simulink model "Quaternions_Method_main"  (R2021b)
settings: Solver=ode4  StartTime=0.0  StopTime=Time  FixedStep=1e-2  RelTol=1e-13  AbsTol=1e-8
values from neighbouring files (symbols this model uses):
  a = 8.6251e+06    (= 8625100)    [Main.m]
  c = 299792*10^3    (= 299792000)    [Main.m]
  e = 0.1195    [Main.m]
  f_mag = 18    [Main.m]
  H_0 = sqrt((g_1_0)^2 + (g_1_1)^2 + (h_1_1)^2)    [Main.m]
  i = 0.3815    [Main.m]
  MB = [2000; 0.3; 1; 0.12].*1e-2    [Main.m]
  muP = G*Mt    (= 398527110340000)    [Main.m]
  omega_0 = [om_x, om_y, om_z]    [Main.m]
  p_acc = 0.5    [Main.m]
  RD = 0.1*ones(1,10)    [Main.m]
  RS_MB = 0.5    [Main.m]
  RS_SP = 0.1    [Main.m]
  SP = [2000; 0.3; 1; 0.12].*1e-2    [Main.m]
  theta0 = 0    [Main.m]
  w_E = (2*pi)/(24*3600)    (= 7.27220521664e-05)    [Main.m]
undefined symbols (not defined in the file or in its folder): A_BN_0, A_rw, A_rw_star, k1, k2, magnitude, mr, sig_b, sig_n, T, t_sample
libraries: matrix_library x15, vrlib x8, simulink x2, simulink_extras x1
(part 3 of 5)

== system Quaternions_Method_main/Enviroment/Magnetic torque /Magnetic torque in body frame/Direction of M field ==
  Clock : Clock
  Constant : Constant  Value=eps
  Constant1 : Constant  Value=w_E
  Mux : Mux  Inputs=3
  Product : Product
  Product1 : Product
  Product2 : Product
  Reshape : Reshape  OutputDimensionality=Column vector (2-D)
  Trigonometric Function : Trigonometry
  Trigonometric Function1 : Trigonometry  Operator=cos
  Trigonometric Function2 : Trigonometry  Operator=cos
  Trigonometric Function3 : Trigonometry
  m_vect : Outport
  wires:
  Constant1/1 -> Product/1
  Clock/1 -> Product/2
  Constant/1 -> Trigonometric Function2/1, Trigonometric Function/1
  Product/1 -> Trigonometric Function3/1, Trigonometric Function1/1
  Trigonometric Function/1 -> Product2/1, Product1/1
  Trigonometric Function1/1 -> Product1/2
  Trigonometric Function3/1 -> Product2/2
  Product1/1 -> Mux/1
  Product2/1 -> Mux/2
  Trigonometric Function2/1 -> Mux/3
  Mux/1 -> Reshape/1
  Reshape/1 -> m_vect/1

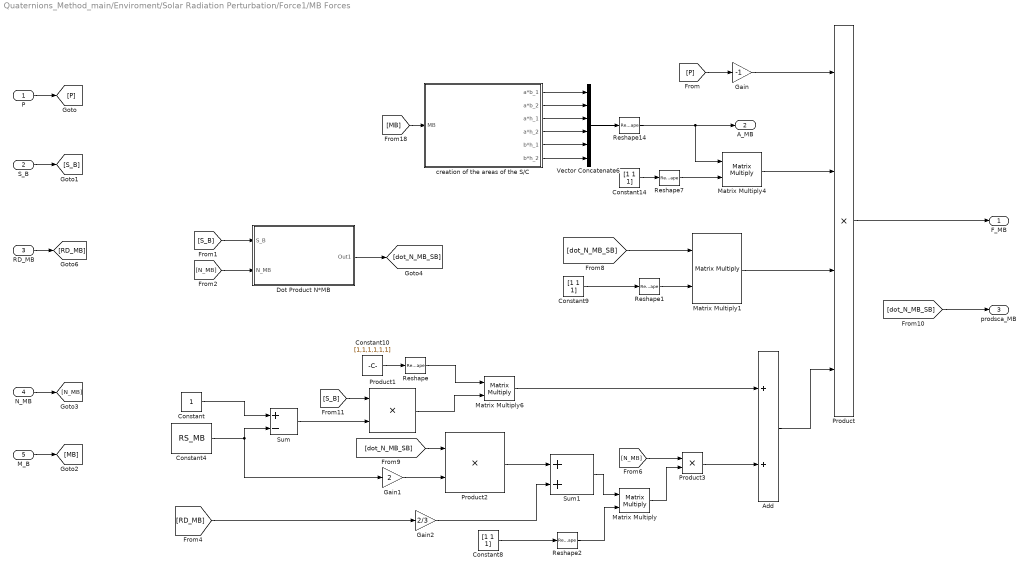
== system Quaternions_Method_main/Enviroment/Solar Radiation Perturbation/Force1/MB Forces ==
  P : Inport
  S_B : Inport  Port=2
  RD_MB : Inport  Port=3
  N_MB : Inport  Port=4
  M_B : Inport  Port=5
  Add : Sum
  Constant : Constant
  Constant10 : Constant  Value=[1,1,1,1,1,1]
  Constant14 : Constant  Value=[1 1 1]
  Constant4 : Constant  Value=RS_MB
  Constant8 : Constant  Value=[1 1 1]
  Constant9 : Constant  Value=[1 1 1]
  Dot Product N*MB : Subsystem
  Gain : Gain  Gain=-1
  Gain1 : Gain  Gain=2
  Gain2 : Gain  Gain=2/3
  Matrix Multiply{,1,4,6} (4 alike) : Product  Multiplication=Matrix(*)
  Product : Product  Inputs=4
  Product1 : Product
  Product2 : Product
  Product3 : Product
  Reshape : Reshape  OutputDimensionality=Column vector (2-D)
  Reshape1 : Reshape  OutputDimensionality=Row vector (2-D)
  Reshape14 : Reshape  OutputDimensionality=Column vector (2-D)
  Reshape2 : Reshape  OutputDimensionality=Row vector (2-D)
  Reshape7 : Reshape  OutputDimensionality=Row vector (2-D)
  Sum : Sum  Inputs=+-
  Sum1 : Sum
  Vector Concatenate6 : Concatenate  NumInputs=6
  creation of the areas of the S/C : Subsystem
  F_MB : Outport
  A_MB : Outport  Port=2
  prodsca_MB : Outport  Port=3
  wires:
  Constant4/1 -> Sum/2, Gain1/1
  Matrix Multiply6/1 -> Add/1
  Vector Concatenate6/1 -> Reshape14/1
  Constant9/1 -> Reshape1/1
  Reshape1/1 -> Matrix Multiply1/2
  Constant/1 -> Sum/1
  Reshape2/1 -> Matrix Multiply/2
  Gain/1 -> Product/1
  [S_B] -> Product1/1
  Sum/1 -> Product1/2
  creation of the areas of the S/C/1(a*b_1) -> Vector Concatenate6/1
  Add/1 -> Product/4
  Constant8/1 -> Reshape2/1
  Gain2/1 -> Sum1/2
  [dot_N_MB_SB] -> prodsca_MB/1
  [RD_MB] -> Gain2/1
  creation of the areas of the S/C/2(a*b_2) -> Vector Concatenate6/2
  [P] -> Gain/1
  Product2/1 -> Sum1/1
  Matrix Multiply/1 -> Product3/2
  [dot_N_MB_SB] -> Matrix Multiply1/1
  Matrix Multiply4/1 -> Product/2
  Reshape14/1 -> A_MB/1, Matrix Multiply4/1
  Matrix Multiply1/1 -> Product/3
  Gain1/1 -> Product2/2
  Sum1/1 -> Matrix Multiply/1
  creation of the areas of the S/C/4(a*h_2) -> Vector Concatenate6/4
  [dot_N_MB_SB] -> Product2/1
  creation of the areas of the S/C/5(b*h_1) -> Vector Concatenate6/5
  creation of the areas of the S/C/6(b*h_2) -> Vector Concatenate6/6
  Product1/1 -> Matrix Multiply6/2
  creation of the areas of the S/C/3(a*h_1) -> Vector Concatenate6/3
  [MB] -> creation of the areas of the S/C/1(MB)
  Constant14/1 -> Reshape7/1
  Product/1 -> F_MB/1
  Reshape7/1 -> Matrix Multiply4/2
  Product3/1 -> Add/2
  Constant10/1 -> Reshape/1
  Reshape/1 -> Matrix Multiply6/1
  [N_MB] -> Product3/1
  Dot Product N*MB/1(Out1) -> [dot_N_MB_SB]
  S_B/1 -> [S_B]
  RD_MB/1 -> [RD_MB]
  P/1 -> [P]
  N_MB/1 -> [N_MB]
  M_B/1 -> [MB]
  [S_B] -> Dot Product N*MB/1(S_B)
  [N_MB] -> Dot Product N*MB/2(N_MB)

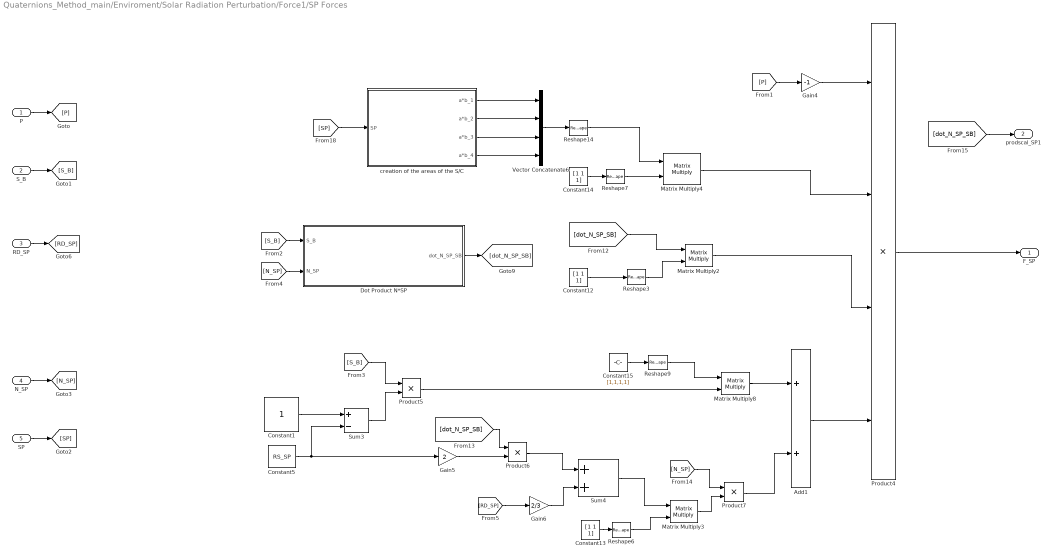
== system Quaternions_Method_main/Enviroment/Solar Radiation Perturbation/Force1/SP Forces ==
  P : Inport
  S_B : Inport  Port=2
  RD_SP : Inport  Port=3
  N_SP : Inport  Port=4
  SP : Inport  Port=5
  Add1 : Sum
  Constant1 : Constant
  Constant12 : Constant  Value=[1 1 1]
  Constant13 : Constant  Value=[1 1 1]
  Constant14 : Constant  Value=[1 1 1]
  Constant15 : Constant  Value=[1,1,1,1]
  Constant5 : Constant  Value=RS_SP
  Dot Product N*SP : Subsystem
  Gain4 : Gain  Gain=-1
  Gain5 : Gain  Gain=2
  Gain6 : Gain  Gain=2/3
  Matrix Multiply{2..4,8} (4 alike) : Product  Multiplication=Matrix(*)
  Product4 : Product  Inputs=4
  Product5 : Product
  Product6 : Product
  Product7 : Product
  Reshape14 : Reshape  OutputDimensionality=Column vector (2-D)
  Reshape3 : Reshape  OutputDimensionality=Row vector (2-D)
  Reshape6 : Reshape  OutputDimensionality=Row vector (2-D)
  Reshape7 : Reshape  OutputDimensionality=Row vector (2-D)
  Reshape9 : Reshape  OutputDimensionality=Column vector (2-D)
  Sum3 : Sum  Inputs=+-
  Sum4 : Sum
  Vector Concatenate6 : Concatenate  NumInputs=4
  creation of the areas of the S/C : Subsystem
  F_SP : Outport
  prodscal_SP1 : Outport  Port=2
  wires:
  Sum3/1 -> Product5/2
  Reshape3/1 -> Matrix Multiply2/2
  Constant13/1 -> Reshape6/1
  Gain4/1 -> Product4/1
  Product6/1 -> Sum4/1
  Constant12/1 -> Reshape3/1
  [S_B] -> Product5/1
  [P] -> Gain4/1
  Gain6/1 -> Sum4/2
  [RD_SP] -> Gain6/1
  [N_SP] -> Product7/1
  Constant1/1 -> Sum3/1
  Constant15/1 -> Reshape9/1
  Sum4/1 -> Matrix Multiply3/1
  Product4/1 -> F_SP/1
  Constant5/1 -> Gain5/1, Sum3/2
  [dot_N_SP_SB] -> Matrix Multiply2/1
  Reshape6/1 -> Matrix Multiply3/2
  Product5/1 -> Matrix Multiply8/2
  Matrix Multiply3/1 -> Product7/2
  Gain5/1 -> Product6/2
  Matrix Multiply2/1 -> Product4/3
  Reshape9/1 -> Matrix Multiply8/1
  Product7/1 -> Add1/2
  [dot_N_SP_SB] -> Product6/1
  Add1/1 -> Product4/4
  [dot_N_SP_SB] -> prodscal_SP1/1
  Matrix Multiply8/1 -> Add1/1
  S_B/1 -> [S_B]
  N_SP/1 -> [N_SP]
  P/1 -> [P]
  SP/1 -> [SP]
  RD_SP/1 -> [RD_SP]
  Matrix Multiply4/1 -> Product4/2
  Vector Concatenate6/1 -> Reshape14/1
  Reshape14/1 -> Matrix Multiply4/1
  Constant14/1 -> Reshape7/1
  [SP] -> creation of the areas of the S/C/1(SP)
  Reshape7/1 -> Matrix Multiply4/2
  creation of the areas of the S/C/1(a*b_1) -> Vector Concatenate6/1
  creation of the areas of the S/C/2(a*b_2) -> Vector Concatenate6/2
  creation of the areas of the S/C/3(a*b_3) -> Vector Concatenate6/3
  creation of the areas of the S/C/4(a*b_4) -> Vector Concatenate6/4
  [S_B] -> Dot Product N*SP/1(S_B)
  [N_SP] -> Dot Product N*SP/2(N_SP)
  Dot Product N*SP/1(dot_N_SP_SB) -> [dot_N_SP_SB]

== system Quaternions_Method_main/Enviroment/Solar Radiation Perturbation/Sum forces/determine highlighted area ==
  note: matrice che ha per colonne i vettori distanza tra il CM del MB e i centri geom delle aree illuminate dal sole
  MB : Inport
  A_MB : Inport  Port=2
  prodscal_MB(tra norm e sun direction) : Inport  Port=3
  Demux1 : Demux  Outputs=6
  Demux2 : Demux  Outputs=6
  If : If  NumInputs=2  IfExpression=u1>0  ElseIfExpressions=u2>0
  If Action Subsystem : Subsystem  TreatAsAtomicUnit=on
  If Action Subsystem1 : Subsystem  TreatAsAtomicUnit=on
  If Action Subsystem2 : Subsystem  TreatAsAtomicUnit=on
  If Action Subsystem3 : Subsystem  TreatAsAtomicUnit=on
  If Action Subsystem4 : Subsystem  TreatAsAtomicUnit=on
  If Action Subsystem5 : Subsystem  TreatAsAtomicUnit=on
  If Action Subsystem6 : Subsystem  TreatAsAtomicUnit=on
  If Action Subsystem7 : Subsystem  TreatAsAtomicUnit=on
  If Action Subsystem8 : Subsystem  TreatAsAtomicUnit=on
  If1 : If  NumInputs=2  IfExpression=u1>0  ElseIfExpressions=u2>0
  If2 : If  NumInputs=2  IfExpression=u1>0  ElseIfExpressions=u2>0
  Merge : Merge  Inputs=3
  Merge1 : Merge  Inputs=3
  Merge2 : Merge  Inputs=3
  Mux : Mux  Inputs=3
  Product{10..15} (6 alike) : Product
  Reshape : Reshape  OutputDimensionality=Column vector (2-D)
  Reshape1 : Reshape  OutputDimensionality=Column vector (2-D)
  "creazione della matrice che ha per colonne i vettori distanza tra il CM del MB e i centri geom delle aree illuminate dal sole " : Subsystem
  distance matrix : Outport
  wires:
  Reshape/1 -> Demux2/1
  prodscal_MB(tra norm e sun direction)/1 -> Reshape/1
  Demux2/1 -> Product15/2  "x"
  Demux2/2 -> Product13/2  "y"
  Demux2/3 -> Product12/2  "z"
  Demux2/4 -> Product11/2  "-x"
  Demux2/5 -> Product10/2  "-y"
  Demux2/6 -> Product14/2  "-z"
  Demux1/1 -> Product12/1
  Mux/1 -> Reshape1/1
  Product15/1 -> If Action Subsystem/1(In1), If/1  "x"
  If/1 -> If Action Subsystem/Action
  Reshape1/1 -> "creazione della matrice che ha per colonne i vettori distanza tra il CM del MB e i centri geom delle aree illuminate dal sole "/2(A_vect)  "Areas_vect = vettore contenente le aree nelle direzioni x, y, z, -x, -y, -z"
  "creazione della matrice che ha per colonne i vettori distanza tra il CM del MB e i centri geom delle aree illuminate dal sole "/1(distance matrix) -> distance matrix/1
  A_MB/1 -> Demux1/1
  Demux1/2 -> Product14/1
  Demux1/3 -> Product13/1
  Demux1/4 -> Product10/1
  Demux1/5 -> Product15/1
  Demux1/6 -> Product11/1
  If/2 -> If Action Subsystem1/Action
  Product11/1 -> If Action Subsystem1/1(In1), If/2  "-x"
  If1/2 -> If Action Subsystem4/Action
  If1/3 -> If Action Subsystem5/Action
  If1/1 -> If Action Subsystem3/Action
  Product10/1 -> If Action Subsystem4/1(In1), If1/2  "-y"
  Product13/1 -> If Action Subsystem3/1(In1), If1/1  "y"
  If2/2 -> If Action Subsystem7/Action
  If2/3 -> If Action Subsystem8/Action
  If2/1 -> If Action Subsystem6/Action
  Product12/1 -> If Action Subsystem6/1(In1), If2/1  "z"
  Product14/1 -> If Action Subsystem7/1(In1), If2/2  "-z"
  Merge/1 -> Mux/2
  Merge2/1 -> Mux/3
  Merge1/1 -> Mux/1
  If Action Subsystem8/1(Out1) -> Merge2/3
  If Action Subsystem7/1(Out1) -> Merge2/2
  If Action Subsystem6/1(Out1) -> Merge2/1
  If Action Subsystem5/1(Out1) -> Merge/3
  If Action Subsystem4/1(Out1) -> Merge/2
  MB/1 -> "creazione della matrice che ha per colonne i vettori distanza tra il CM del MB e i centri geom delle aree illuminate dal sole "/1(MB)
  If Action Subsystem/1(Out1) -> Merge1/1
  If Action Subsystem1/1(Out1) -> Merge1/2
  If/3 -> If Action Subsystem2/Action
  If Action Subsystem2/1(Out1) -> Merge1/3
  If Action Subsystem3/1(Out1) -> Merge/1

== system Quaternions_Method_main/Enviroment/Solar Radiation Perturbation/Sum forces/determine highlighted area1 ==
  prodscal_SP(tra norm e sun direction) : Inport
  Demux2 : Demux
  If : If  NumInputs=2  IfExpression=u1>0  ElseIfExpressions=u2>0
  If Action Subsystem : Subsystem  TreatAsAtomicUnit=on
  If Action Subsystem1 : Subsystem  TreatAsAtomicUnit=on
  If Action Subsystem2 : Subsystem  TreatAsAtomicUnit=on
  If Action Subsystem3 : Subsystem  TreatAsAtomicUnit=on
  If Action Subsystem4 : Subsystem  TreatAsAtomicUnit=on
  If Action Subsystem5 : Subsystem  TreatAsAtomicUnit=on
  If1 : If  NumInputs=2  IfExpression=u1>0  ElseIfExpressions=u2>0
  Merge : Merge  Inputs=3
  Merge1 : Merge  Inputs=3
  Mux : Mux  Inputs=2
  Reshape : Reshape  OutputDimensionality=Column vector (2-D)
  Reshape1 : Reshape  OutputDimensionality=Column vector (2-D)
  face illuminated : Outport
  wires:
  If Action Subsystem2/1(Out1) -> Merge/3
  If/3 -> If Action Subsystem2/Action
  Merge/1 -> Mux/1
  Demux2/1 -> If/1  "y_1"
  Mux/1 -> Reshape1/1
  Demux2/2 -> If/2  "-y_1"
  prodscal_SP(tra norm e sun direction)/1 -> Reshape/1
  Reshape/1 -> Demux2/1
  Demux2/3 -> If1/1  "y_2"
  Demux2/4 -> If1/2  "-y_2"
  Merge1/1 -> Mux/2
  Reshape1/1 -> face illuminated/1
  If/1 -> If Action Subsystem/Action
  If Action Subsystem/1(Out1) -> Merge/1
  If/2 -> If Action Subsystem1/Action
  If Action Subsystem1/1(Out1) -> Merge/2
  If Action Subsystem4/1(Out1) -> Merge1/2
  If1/2 -> If Action Subsystem4/Action
  If1/1 -> If Action Subsystem3/Action
  If1/3 -> If Action Subsystem5/Action
  If Action Subsystem5/1(Out1) -> Merge1/3
  If Action Subsystem3/1(Out1) -> Merge1/1

== system Quaternions_Method_main/Kinematics1/Creazione quaternione/DCM to quaternion/Case 1 ==
  A11 : Inport
  A22 : Inport  Port=2
  A33 : Inport  Port=3
  Add : Sum  Inputs=++--
  Constant : Constant
  Gain : Gain  Gain=1/2
  Sqrt : Sqrt  SaturateOnIntegerOverflow=on
  q1 : Outport
  wires:
  A22/1 -> Add/3
  A11/1 -> Add/2
  A33/1 -> Add/4
  Constant/1 -> Add/1
  Add/1 -> Sqrt/1
  Sqrt/1 -> Gain/1
  Gain/1 -> q1/1

== system Quaternions_Method_main/Kinematics1/Creazione quaternione/DCM to quaternion/Case 2 ==
  A11 : Inport
  A22 : Inport  Port=2
  A33 : Inport  Port=3
  Add : Sum  Inputs=+-+-
  Constant : Constant
  Gain : Gain  Gain=1/2
  Sqrt : Sqrt  SaturateOnIntegerOverflow=on
  q2 : Outport
  wires:
  Gain/1 -> q2/1
  Sqrt/1 -> Gain/1
  Add/1 -> Sqrt/1
  Constant/1 -> Add/1
  A33/1 -> Add/4
  A11/1 -> Add/2
  A22/1 -> Add/3

== system Quaternions_Method_main/Kinematics1/Creazione quaternione/DCM to quaternion/Case 3 ==
  A11 : Inport
  A22 : Inport  Port=2
  A33 : Inport  Port=3
  Add : Sum  Inputs=+--+
  Constant : Constant
  Gain : Gain  Gain=1/2
  Sqrt : Sqrt  SaturateOnIntegerOverflow=on
  q3 : Outport
  wires:
  A22/1 -> Add/3
  A11/1 -> Add/2
  A33/1 -> Add/4
  Constant/1 -> Add/1
  Add/1 -> Sqrt/1
  Sqrt/1 -> Gain/1
  Gain/1 -> q3/1

== system Quaternions_Method_main/Kinematics1/Creazione quaternione/DCM to quaternion/Case 4 ==
  A11 : Inport
  A22 : Inport  Port=2
  A33 : Inport  Port=3
  Add : Sum  Inputs=++++
  Constant : Constant
  Gain : Gain  Gain=1/2
  Sqrt : Sqrt  SaturateOnIntegerOverflow=on
  q4 : Outport
  wires:
  Gain/1 -> q4/1
  Sqrt/1 -> Gain/1
  Add/1 -> Sqrt/1
  Constant/1 -> Add/1
  A33/1 -> Add/4
  A11/1 -> Add/2
  A22/1 -> Add/3

== system Quaternions_Method_main/Kinematics1/Creazione quaternione/DCM to quaternion/If Action Subsystem ==
  In2 : Inport
  In1 : Inport  Port=2
  Action Port : ActionPort  ActionPortLabel=if(u1 == u2)
  Add : Sum
  Add1 : Sum
  Add2 : Sum  Inputs=+-
  Demux : Demux  Outputs=6
  Gain : Gain  Gain=4
  Mux : Mux
  Product : Product
  Product1 : Product
  Product2 : Product
  Reciprocal : Product  Inputs=/
  Reshape : Reshape  OutputDimensionality=Column vector (2-D)
  q_vect1 : Outport
  wires:
  In1/1 -> Demux/1
  In2/1 -> [q1]
  Mux/1 -> Reshape/1
  Reshape/1 -> q_vect1/1
  [q1] -> Mux/1
  Demux/3 -> [A12]
  Demux/2 -> [A31]
  Demux/1 -> [A21]
  Demux/6 -> [A23]
  Demux/5 -> [A13]
  Demux/4 -> [A32]
  [q1] -> Gain/1
  Gain/1 -> Reciprocal/1
  Reciprocal/1 -> [q1_div]
  Add/1 -> Product/1
  [A21] -> Add/2
  [A12] -> Add/1
  [q1_div] -> Product/2
  Product/1 -> [q2]
  Product1/1 -> [q3]
  [q1_div] -> Product1/2
  [A13] -> Add1/1
  [A31] -> Add1/2
  Add1/1 -> Product1/1
  Add2/1 -> Product2/1
  [A32] -> Add2/2
  [A23] -> Add2/1
  [q1_div] -> Product2/2
  Product2/1 -> [q4]
  [q2] -> Mux/2
  [q3] -> Mux/3
  [q4] -> Mux/4

== system Quaternions_Method_main/Kinematics1/Creazione quaternione/DCM to quaternion/If Action Subsystem1 ==
  In2 : Inport
  In1 : Inport  Port=2
  Action Port : ActionPort  ActionPortLabel=elseif(u1 == u3)
  Add : Sum
  Add1 : Sum  Inputs=-+
  Add2 : Sum
  Demux : Demux  Outputs=6
  Gain : Gain  Gain=4
  Mux : Mux
  Product : Product
  Product1 : Product
  Product2 : Product
  Reciprocal : Product  Inputs=/
  Reshape : Reshape  OutputDimensionality=Column vector (2-D)
  q_vect2 : Outport
  wires:
  [q4] -> Mux/4
  [q3] -> Mux/3
  [q2] -> Mux/2
  Product2/1 -> [q3]
  [q2_div] -> Product2/2
  [A23] -> Add2/1
  [A32] -> Add2/2
  Add2/1 -> Product2/1
  Add1/1 -> Product1/1
  [A31] -> Add1/2
  [A13] -> Add1/1
  [q2_div] -> Product1/2
  Product1/1 -> [q4]
  Product/1 -> [q1]
  [q2_div] -> Product/2
  [A12] -> Add/1
  [A21] -> Add/2
  Add/1 -> Product/1
  Reciprocal/1 -> [q2_div]
  Gain/1 -> Reciprocal/1
  [q2] -> Gain/1
  Demux/4 -> [A32]
  Demux/5 -> [A13]
  Demux/6 -> [A23]
  Demux/1 -> [A21]
  Demux/2 -> [A31]
  Demux/3 -> [A12]
  [q1] -> Mux/1
  Reshape/1 -> q_vect2/1
  Mux/1 -> Reshape/1
  In2/1 -> [q2]
  In1/1 -> Demux/1

== system Quaternions_Method_main/Kinematics1/Creazione quaternione/DCM to quaternion/If Action Subsystem2 ==
  In2 : Inport
  In1 : Inport  Port=2
  Action Port : ActionPort  ActionPortLabel=elseif( u1 == u4)
  Add : Sum  Inputs=+-
  Add1 : Sum
  Add2 : Sum  Inputs=+-
  Demux : Demux  Outputs=6
  Gain : Gain  Gain=4
  Mux : Mux
  Product : Product
  Product1 : Product
  Product2 : Product
  Reciprocal : Product  Inputs=/
  Reshape : Reshape  OutputDimensionality=Column vector (2-D)
  q_vect3 : Outport
  wires:
  In1/1 -> Demux/1
  In2/1 -> [q3]
  Mux/1 -> Reshape/1
  Reshape/1 -> q_vect3/1
  [q1] -> Mux/1
  Demux/3 -> [A12]
  Demux/2 -> [A31]
  Demux/1 -> [A21]
  Demux/6 -> [A23]
  Demux/5 -> [A13]
  Demux/4 -> [A32]
  [q3] -> Gain/1
  Gain/1 -> Reciprocal/1
  Reciprocal/1 -> [q3_div]
  Add/1 -> Product/1
  [A21] -> Add/2
  [A12] -> Add/1
  [q3_div] -> Product/2
  Product/1 -> [q4]
  Product1/1 -> [q1]
  [q3_div] -> Product1/2
  [A13] -> Add1/1
  [A31] -> Add1/2
  Add1/1 -> Product1/1
  Add2/1 -> Product2/1
  [A32] -> Add2/2
  [A23] -> Add2/1
  [q3_div] -> Product2/2
  Product2/1 -> [q2]
  [q2] -> Mux/2
  [q3] -> Mux/3
  [q4] -> Mux/4

== system Quaternions_Method_main/Kinematics1/Creazione quaternione/DCM to quaternion/If Action Subsystem3 ==
  In2 : Inport
  In1 : Inport  Port=2
  Action Port : ActionPort  ActionPortLabel=elseif( u1 == u5)
  Add : Sum  Inputs=+-
  Add1 : Sum  Inputs=-+
  Add2 : Sum  Inputs=+-
  Demux : Demux  Outputs=6
  Gain : Gain  Gain=4
  Mux : Mux
  Product : Product
  Product1 : Product
  Product2 : Product
  Reciprocal : Product  Inputs=/
  Reshape : Reshape  OutputDimensionality=Column vector (2-D)
  q_vect4 : Outport
  wires:
  [q4] -> Mux/4
  [q3] -> Mux/3
  [q2] -> Mux/2
  Product2/1 -> [q1]
  [q4_div] -> Product2/2
  [A23] -> Add2/1
  [A32] -> Add2/2
  Add2/1 -> Product2/1
  Add1/1 -> Product1/1
  [A31] -> Add1/2
  [A13] -> Add1/1
  [q4_div] -> Product1/2
  Product1/1 -> [q2]
  Product/1 -> [q3]
  [q4_div] -> Product/2
  [A12] -> Add/1
  [A21] -> Add/2
  Add/1 -> Product/1
  Reciprocal/1 -> [q4_div]
  Gain/1 -> Reciprocal/1
  [q4] -> Gain/1
  Demux/4 -> [A32]
  Demux/5 -> [A13]
  Demux/6 -> [A23]
  Demux/1 -> [A21]
  Demux/2 -> [A31]
  Demux/3 -> [A12]
  [q1] -> Mux/1
  Reshape/1 -> q_vect4/1
  Mux/1 -> Reshape/1
  In2/1 -> [q4]
  In1/1 -> Demux/1

== system Quaternions_Method_main/Kinematics1/Relative_Attitude/A_LN/M1 ==
  Input : Inport
  Constant{1..2,4..5} (4 alike) : Constant  Value=0
  Constant3 : Constant
  Cos : Trigonometry  Operator=cos
  Cos1 : Trigonometry
  Cos2 : Trigonometry  Operator=cos
  Cos3 : Trigonometry
  Matrix Concatenate : Concatenate  NumInputs=3  Mode=Multidimensional array  ConcatenateDimension=2
  Multiply : Gain  Gain=-1
  Mux : Mux  Inputs=3
  Mux1 : Mux  Inputs=3
  Mux2 : Mux  Inputs=3
  Reshape : Reshape  OutputDimensionality=Column vector (2-D)
  Reshape1 : Reshape  OutputDimensionality=Column vector (2-D)
  Reshape2 : Reshape  OutputDimensionality=Column vector (2-D)
  Out1 : Outport
  wires:
  Multiply/1 -> Mux/2
  Cos/1 -> Mux/1
  Constant1/1 -> Mux/3
  Constant2/1 -> Mux1/3
  Input/1 -> Cos/1, Cos1/1, Cos3/1, Cos2/1
  Matrix Concatenate/1 -> Out1/1
  Cos3/1 -> Mux1/1
  Constant5/1 -> Mux2/1
  Cos2/1 -> Mux1/2
  Constant3/1 -> Mux2/3
  Constant4/1 -> Mux2/2
  Cos1/1 -> Multiply/1
  Mux/1 -> Reshape/1
  Reshape/1 -> Matrix Concatenate/1
  Reshape1/1 -> Matrix Concatenate/2
  Mux1/1 -> Reshape1/1
  Mux2/1 -> Reshape2/1
  Reshape2/1 -> Matrix Concatenate/3

== system Quaternions_Method_main/Kinematics1/Relative_Attitude/A_LN/M2 ==
  ii : Inport
  Constant{1..4} (4 alike) : Constant  Value=0
  Constant5 : Constant
  Cos : Trigonometry  Operator=cos
  Cos1 : Trigonometry
  Cos2 : Trigonometry  Operator=cos
  Cos3 : Trigonometry
  Matrix Concatenate : Concatenate  NumInputs=3  Mode=Multidimensional array  ConcatenateDimension=2
  Multiply : Gain  Gain=-1
  Mux : Mux  Inputs=3
  Mux1 : Mux  Inputs=3
  Mux2 : Mux  Inputs=3
  Reshape : Reshape  OutputDimensionality=Column vector (2-D)
  Reshape1 : Reshape  OutputDimensionality=Column vector (2-D)
  Reshape2 : Reshape  OutputDimensionality=Column vector (2-D)
  Out1 : Outport
  wires:
  Matrix Concatenate/1 -> Out1/1
  Constant5/1 -> Mux2/1
  Constant3/1 -> Mux2/3
  Constant4/1 -> Mux2/2
  Cos1/1 -> Multiply/1
  Constant1/1 -> Mux/1
  Cos/1 -> Mux/2
  Multiply/1 -> Mux/3
  Constant2/1 -> Mux1/1
  Cos3/1 -> Mux1/2
  Cos2/1 -> Mux1/3
  ii/1 -> Cos2/1, Cos/1, Cos1/1, Cos3/1
  Mux2/1 -> Reshape/1
  Reshape/1 -> Matrix Concatenate/1
  Mux/1 -> Reshape1/1
  Reshape1/1 -> Matrix Concatenate/2
  Reshape2/1 -> Matrix Concatenate/3
  Mux1/1 -> Reshape2/1

== system Quaternions_Method_main/Sensors/Magnetometer1/Magnetometer /Error Matrices ==
  A_NonOrtho : Subsystem
  A_ScaleFactor : Subsystem
  A_eps : Subsystem
  A_no : Outport
  A_sf : Outport  Port=2
  A_noise : Outport  Port=3
  wires:
  A_NonOrtho/1(A_no) -> A_no/1
  A_ScaleFactor/1(A_sf) -> A_sf/1
  A_eps/1(A_eps) -> A_noise/1

== system Quaternions_Method_main/Sensors/Magnetometer1/Magnetometer /RC Low Pass FIlter ==
  A* : Inport
  Add : Sum  Inputs=||+||-||
  Discrete Derivative : simulink/Discrete/Discrete Derivative  gainval=10  ICPrevScaledInput=0.0  OutMin=[]  OutMax=[]  OutDataType=fixdt(1, 16)  OutScaling=2^-10  DoSatur=off
  A*_filtered : Outport
  wires:
  A*/1 -> Add/1
  Add/1 -> Discrete Derivative/1, A*_filtered/1
  Discrete Derivative/1 -> Add/2

== system Quaternions_Method_main/Sensors/Magnetometer1/Magnetometer /orthonormalization step 1 ==
  A*(t) : Inport
  Gain : Gain  Gain=3/2
  Gain1 : Gain  Gain=1/2
  Matrix Multiply : Product  Inputs=3  Multiplication=Matrix(*)
  Sum : Sum  Inputs=-+
  Transpose : Math  Operator=transpose  SaturateOnIntegerOverflow=on
  A_BN*_filtered : Outport
  wires:
  A*(t)/1 -> Transpose/1, Gain1/1, Matrix Multiply/1, Gain/1
  Sum/1 -> A_BN*_filtered/1
  Gain/1 -> Sum/2
  Transpose/1 -> Matrix Multiply/2
  Gain1/1 -> Matrix Multiply/3
  Matrix Multiply/1 -> Sum/1

== system Quaternions_Method_main/Sensors/Magnetometer1/Magnetometer /orthonormalization step 2 ==
  A*(t) : Inport
  Gain : Gain  Gain=3/2
  Gain1 : Gain  Gain=1/2
  Matrix Multiply : Product  Inputs=3  Multiplication=Matrix(*)
  Sum : Sum  Inputs=-+
  Transpose : Math  Operator=transpose  SaturateOnIntegerOverflow=on
  A_BN*_filtered : Outport
  wires:
  Matrix Multiply/1 -> Sum/1
  Gain1/1 -> Matrix Multiply/3
  Transpose/1 -> Matrix Multiply/2
  Gain/1 -> Sum/2
  Sum/1 -> A_BN*_filtered/1
  A*(t)/1 -> Gain/1, Matrix Multiply/1, Gain1/1, Transpose/1

== system Quaternions_Method_main/Sensors/Magnetometer1/Magnetometer /orthonormalization step 3 ==
  A*(t) : Inport
  Gain : Gain  Gain=3/2
  Gain1 : Gain  Gain=1/2
  Matrix Multiply : Product  Inputs=3  Multiplication=Matrix(*)
  Sum : Sum  Inputs=-+
  Transpose : Math  Operator=transpose  SaturateOnIntegerOverflow=on
  A_BN*_filtered : Outport
  wires:
  A*(t)/1 -> Transpose/1, Gain1/1, Matrix Multiply/1, Gain/1
  Sum/1 -> A_BN*_filtered/1
  Gain/1 -> Sum/2
  Transpose/1 -> Matrix Multiply/2
  Gain1/1 -> Matrix Multiply/3
  Matrix Multiply/1 -> Sum/1

== system Quaternions_Method_main/Sensors/Magnetometer1/b_B computation/Saturation ==
  b_B : Inport
  Dot Product : DotProduct  InputSameDT=on  OutDataTypeStr=Inherit: Inherit via internal rule
  If : If  NumInputs=2  IfExpression=u1 < mr
  If Action Subsystem : Subsystem  TreatAsAtomicUnit=on
  If Action Subsystem1 : Subsystem  TreatAsAtomicUnit=on
  Merge : Merge
  Square Root : Sqrt  SaturateOnIntegerOverflow=on
  measurament range : Constant  Value=mr
  b_B saturated : Outport
  wires:
  b_B/1 -> If Action Subsystem1/2(b_B), Dot Product/2, If Action Subsystem/1(b_B), Dot Product/1
  Dot Product/1 -> Square Root/1
  If Action Subsystem/1(b_B*) -> Merge/1
  If/1 -> If Action Subsystem/Action
  If Action Subsystem1/1(b_B_sat) -> Merge/2
  If/2 -> If Action Subsystem1/Action
  Square Root/1 -> If/1
  measurament range/1 -> If Action Subsystem1/1(mr), If/2
  Merge/1 -> b_B saturated/1

== system Quaternions_Method_main/Sun Pointing 1/Pointing error with quaternions/A_B_N from Euler to quaternion/Case 1 ==
  A11 : Inport
  A22 : Inport  Port=2
  A33 : Inport  Port=3
  Add : Sum  Inputs=++--
  Constant : Constant
  Gain : Gain  Gain=1/2
  Sqrt : Sqrt  SaturateOnIntegerOverflow=on
  q1 : Outport
  wires:
  A22/1 -> Add/3
  A11/1 -> Add/2
  A33/1 -> Add/4
  Constant/1 -> Add/1
  Add/1 -> Sqrt/1
  Sqrt/1 -> Gain/1
  Gain/1 -> q1/1

== system Quaternions_Method_main/Sun Pointing 1/Pointing error with quaternions/A_B_N from Euler to quaternion/Case 2 ==
  A11 : Inport
  A22 : Inport  Port=2
  A33 : Inport  Port=3
  Add : Sum  Inputs=+-+-
  Constant : Constant
  Gain : Gain  Gain=1/2
  Sqrt : Sqrt  SaturateOnIntegerOverflow=on
  q2 : Outport
  wires:
  Gain/1 -> q2/1
  Sqrt/1 -> Gain/1
  Add/1 -> Sqrt/1
  Constant/1 -> Add/1
  A33/1 -> Add/4
  A11/1 -> Add/2
  A22/1 -> Add/3

== system Quaternions_Method_main/Sun Pointing 1/Pointing error with quaternions/A_B_N from Euler to quaternion/Case 3 ==
  A11 : Inport
  A22 : Inport  Port=2
  A33 : Inport  Port=3
  Add : Sum  Inputs=+--+
  Constant : Constant
  Gain : Gain  Gain=1/2
  Sqrt : Sqrt  SaturateOnIntegerOverflow=on
  q3 : Outport
  wires:
  A22/1 -> Add/3
  A11/1 -> Add/2
  A33/1 -> Add/4
  Constant/1 -> Add/1
  Add/1 -> Sqrt/1
  Sqrt/1 -> Gain/1
  Gain/1 -> q3/1

== system Quaternions_Method_main/Sun Pointing 1/Pointing error with quaternions/A_B_N from Euler to quaternion/Case 4 ==
  A11 : Inport
  A22 : Inport  Port=2
  A33 : Inport  Port=3
  Add : Sum  Inputs=++++
  Constant : Constant
  Gain : Gain  Gain=1/2
  Sqrt : Sqrt  SaturateOnIntegerOverflow=on
  q4 : Outport
  wires:
  Gain/1 -> q4/1
  Sqrt/1 -> Gain/1
  Add/1 -> Sqrt/1
  Constant/1 -> Add/1
  A33/1 -> Add/4
  A11/1 -> Add/2
  A22/1 -> Add/3

== system Quaternions_Method_main/Sun Pointing 1/Pointing error with quaternions/A_B_N from Euler to quaternion/If Action Subsystem ==
  In2 : Inport
  In1 : Inport  Port=2
  Action Port : ActionPort  ActionPortLabel=if(u1 == u2)
  Add : Sum
  Add1 : Sum
  Add2 : Sum  Inputs=+-
  Demux : Demux  Outputs=6
  Gain : Gain  Gain=4
  Mux : Mux
  Product : Product
  Product1 : Product
  Product2 : Product
  Reciprocal : Product  Inputs=/
  Reshape : Reshape  OutputDimensionality=Column vector (2-D)
  q_vect1 : Outport
  wires:
  In1/1 -> Demux/1
  In2/1 -> [q1]
  Mux/1 -> Reshape/1
  Reshape/1 -> q_vect1/1
  [q1] -> Mux/1
  Demux/3 -> [A12]
  Demux/2 -> [A31]
  Demux/1 -> [A21]
  Demux/6 -> [A23]
  Demux/5 -> [A13]
  Demux/4 -> [A32]
  [q1] -> Gain/1
  Gain/1 -> Reciprocal/1
  Reciprocal/1 -> [q1_div]
  Add/1 -> Product/1
  [A21] -> Add/2
  [A12] -> Add/1
  [q1_div] -> Product/2
  Product/1 -> [q2]
  Product1/1 -> [q3]
  [q1_div] -> Product1/2
  [A13] -> Add1/1
  [A31] -> Add1/2
  Add1/1 -> Product1/1
  Add2/1 -> Product2/1
  [A32] -> Add2/2
  [A23] -> Add2/1
  [q1_div] -> Product2/2
  Product2/1 -> [q4]
  [q2] -> Mux/2
  [q3] -> Mux/3
  [q4] -> Mux/4

== system Quaternions_Method_main/Sun Pointing 1/Pointing error with quaternions/A_B_N from Euler to quaternion/If Action Subsystem1 ==
  In2 : Inport
  In1 : Inport  Port=2
  Action Port : ActionPort  ActionPortLabel=elseif(u1 == u3)
  Add : Sum
  Add1 : Sum  Inputs=-+
  Add2 : Sum
  Demux : Demux  Outputs=6
  Gain : Gain  Gain=4
  Mux : Mux
  Product : Product
  Product1 : Product
  Product2 : Product
  Reciprocal : Product  Inputs=/
  Reshape : Reshape  OutputDimensionality=Column vector (2-D)
  q_vect2 : Outport
  wires:
  [q4] -> Mux/4
  [q3] -> Mux/3
  [q2] -> Mux/2
  Product2/1 -> [q3]
  [q2_div] -> Product2/2
  [A23] -> Add2/1
  [A32] -> Add2/2
  Add2/1 -> Product2/1
  Add1/1 -> Product1/1
  [A31] -> Add1/2
  [A13] -> Add1/1
  [q2_div] -> Product1/2
  Product1/1 -> [q4]
  Product/1 -> [q1]
  [q2_div] -> Product/2
  [A12] -> Add/1
  [A21] -> Add/2
  Add/1 -> Product/1
  Reciprocal/1 -> [q2_div]
  Gain/1 -> Reciprocal/1
  [q2] -> Gain/1
  Demux/4 -> [A32]
  Demux/5 -> [A13]
  Demux/6 -> [A23]
  Demux/1 -> [A21]
  Demux/2 -> [A31]
  Demux/3 -> [A12]
  [q1] -> Mux/1
  Reshape/1 -> q_vect2/1
  Mux/1 -> Reshape/1
  In2/1 -> [q2]
  In1/1 -> Demux/1

== system Quaternions_Method_main/Sun Pointing 1/Pointing error with quaternions/A_B_N from Euler to quaternion/If Action Subsystem2 ==
  In2 : Inport
  In1 : Inport  Port=2
  Action Port : ActionPort  ActionPortLabel=elseif( u1 == u4)
  Add : Sum  Inputs=+-
  Add1 : Sum
  Add2 : Sum  Inputs=+-
  Demux : Demux  Outputs=6
  Gain : Gain  Gain=4
  Mux : Mux
  Product : Product
  Product1 : Product
  Product2 : Product
  Reciprocal : Product  Inputs=/
  Reshape : Reshape  OutputDimensionality=Column vector (2-D)
  q_vect3 : Outport
  wires:
  In1/1 -> Demux/1
  In2/1 -> [q3]
  Mux/1 -> Reshape/1
  Reshape/1 -> q_vect3/1
  [q1] -> Mux/1
  Demux/3 -> [A12]
  Demux/2 -> [A31]
  Demux/1 -> [A21]
  Demux/6 -> [A23]
  Demux/5 -> [A13]
  Demux/4 -> [A32]
  [q3] -> Gain/1
  Gain/1 -> Reciprocal/1
  Reciprocal/1 -> [q3_div]
  Add/1 -> Product/1
  [A21] -> Add/2
  [A12] -> Add/1
  [q3_div] -> Product/2
  Product/1 -> [q4]
  Product1/1 -> [q1]
  [q3_div] -> Product1/2
  [A13] -> Add1/1
  [A31] -> Add1/2
  Add1/1 -> Product1/1
  Add2/1 -> Product2/1
  [A32] -> Add2/2
  [A23] -> Add2/1
  [q3_div] -> Product2/2
  Product2/1 -> [q2]
  [q2] -> Mux/2
  [q3] -> Mux/3
  [q4] -> Mux/4

== system Quaternions_Method_main/Sun Pointing 1/Pointing error with quaternions/A_B_N from Euler to quaternion/If Action Subsystem3 ==
  In2 : Inport
  In1 : Inport  Port=2
  Action Port : ActionPort  ActionPortLabel=elseif( u1 == u5)
  Add : Sum  Inputs=+-
  Add1 : Sum  Inputs=-+
  Add2 : Sum  Inputs=+-
  Demux : Demux  Outputs=6
  Gain : Gain  Gain=4
  Mux : Mux
  Product : Product
  Product1 : Product
  Product2 : Product
  Reciprocal : Product  Inputs=/
  Reshape : Reshape  OutputDimensionality=Column vector (2-D)
  q_vect4 : Outport
  wires:
  [q4] -> Mux/4
  [q3] -> Mux/3
  [q2] -> Mux/2
  Product2/1 -> [q1]
  [q4_div] -> Product2/2
  [A23] -> Add2/1
  [A32] -> Add2/2
  Add2/1 -> Product2/1
  Add1/1 -> Product1/1
  [A31] -> Add1/2
  [A13] -> Add1/1
  [q4_div] -> Product1/2
  Product1/1 -> [q2]
  Product/1 -> [q3]
  [q4_div] -> Product/2
  [A12] -> Add/1
  [A21] -> Add/2
  Add/1 -> Product/1
  Reciprocal/1 -> [q4_div]
  Gain/1 -> Reciprocal/1
  [q4] -> Gain/1
  Demux/4 -> [A32]
  Demux/5 -> [A13]
  Demux/6 -> [A23]
  Demux/1 -> [A21]
  Demux/2 -> [A31]
  Demux/3 -> [A12]
  [q1] -> Mux/1
  Reshape/1 -> q_vect4/1
  Mux/1 -> Reshape/1
  In2/1 -> [q4]
  In1/1 -> Demux/1

== system Quaternions_Method_main/Sun Pointing 1/Pointing error with quaternions/A_B_N from attitude det to quaternion2/Case 1 ==
  A11 : Inport
  A22 : Inport  Port=2
  A33 : Inport  Port=3
  Add : Sum  Inputs=++--
  Constant : Constant
  Gain : Gain  Gain=1/2
  Sqrt : Sqrt  SaturateOnIntegerOverflow=on
  q1 : Outport
  wires:
  Gain/1 -> q1/1
  Sqrt/1 -> Gain/1
  Add/1 -> Sqrt/1
  Constant/1 -> Add/1
  A33/1 -> Add/4
  A11/1 -> Add/2
  A22/1 -> Add/3

== system Quaternions_Method_main/Sun Pointing 1/Pointing error with quaternions/A_B_N from attitude det to quaternion2/Case 2 ==
  A11 : Inport
  A22 : Inport  Port=2
  A33 : Inport  Port=3
  Add : Sum  Inputs=+-+-
  Constant : Constant
  Gain : Gain  Gain=1/2
  Sqrt : Sqrt  SaturateOnIntegerOverflow=on
  q2 : Outport
  wires:
  A22/1 -> Add/3
  A11/1 -> Add/2
  A33/1 -> Add/4
  Constant/1 -> Add/1
  Add/1 -> Sqrt/1
  Sqrt/1 -> Gain/1
  Gain/1 -> q2/1

== system Quaternions_Method_main/Sun Pointing 1/Pointing error with quaternions/A_B_N from attitude det to quaternion2/Case 3 ==
  A11 : Inport
  A22 : Inport  Port=2
  A33 : Inport  Port=3
  Add : Sum  Inputs=+--+
  Constant : Constant
  Gain : Gain  Gain=1/2
  Sqrt : Sqrt  SaturateOnIntegerOverflow=on
  q3 : Outport
  wires:
  Gain/1 -> q3/1
  Sqrt/1 -> Gain/1
  Add/1 -> Sqrt/1
  Constant/1 -> Add/1
  A33/1 -> Add/4
  A11/1 -> Add/2
  A22/1 -> Add/3

== system Quaternions_Method_main/Sun Pointing 1/Pointing error with quaternions/A_B_N from attitude det to quaternion2/Case 4 ==
  A11 : Inport
  A22 : Inport  Port=2
  A33 : Inport  Port=3
  Add : Sum  Inputs=++++
  Constant : Constant
  Gain : Gain  Gain=1/2
  Sqrt : Sqrt  SaturateOnIntegerOverflow=on
  q4 : Outport
  wires:
  A22/1 -> Add/3
  A11/1 -> Add/2
  A33/1 -> Add/4
  Constant/1 -> Add/1
  Add/1 -> Sqrt/1
  Sqrt/1 -> Gain/1
  Gain/1 -> q4/1

== system Quaternions_Method_main/Sun Pointing 1/Pointing error with quaternions/A_B_N from attitude det to quaternion2/If Action Subsystem ==
  In2 : Inport
  In1 : Inport  Port=2
  Action Port : ActionPort  ActionPortLabel=if(u1 == u2)
  Add : Sum
  Add1 : Sum
  Add2 : Sum  Inputs=+-
  Demux : Demux  Outputs=6
  Gain : Gain  Gain=4
  Mux : Mux
  Product : Product
  Product1 : Product
  Product2 : Product
  Reciprocal : Product  Inputs=/
  Reshape : Reshape  OutputDimensionality=Column vector (2-D)
  q_vect1 : Outport
  wires:
  [q4] -> Mux/4
  [q3] -> Mux/3
  [q2] -> Mux/2
  Product2/1 -> [q4]
  [q1_div] -> Product2/2
  [A23] -> Add2/1
  [A32] -> Add2/2
  Add2/1 -> Product2/1
  Add1/1 -> Product1/1
  [A31] -> Add1/2
  [A13] -> Add1/1
  [q1_div] -> Product1/2
  Product1/1 -> [q3]
  Product/1 -> [q2]
  [q1_div] -> Product/2
  [A12] -> Add/1
  [A21] -> Add/2
  Add/1 -> Product/1
  Reciprocal/1 -> [q1_div]
  Gain/1 -> Reciprocal/1
  [q1] -> Gain/1
  Demux/4 -> [A32]
  Demux/5 -> [A13]
  Demux/6 -> [A23]
  Demux/1 -> [A21]
  Demux/2 -> [A31]
  Demux/3 -> [A12]
  [q1] -> Mux/1
  Reshape/1 -> q_vect1/1
  Mux/1 -> Reshape/1
  In2/1 -> [q1]
  In1/1 -> Demux/1

== system Quaternions_Method_main/Sun Pointing 1/Pointing error with quaternions/A_B_N from attitude det to quaternion2/If Action Subsystem1 ==
  In2 : Inport
  In1 : Inport  Port=2
  Action Port : ActionPort  ActionPortLabel=elseif(u1 == u3)
  Add : Sum
  Add1 : Sum  Inputs=-+
  Add2 : Sum
  Demux : Demux  Outputs=6
  Gain : Gain  Gain=4
  Mux : Mux
  Product : Product
  Product1 : Product
  Product2 : Product
  Reciprocal : Product  Inputs=/
  Reshape : Reshape  OutputDimensionality=Column vector (2-D)
  q_vect2 : Outport
  wires:
  In1/1 -> Demux/1
  In2/1 -> [q2]
  Mux/1 -> Reshape/1
  Reshape/1 -> q_vect2/1
  [q1] -> Mux/1
  Demux/3 -> [A12]
  Demux/2 -> [A31]
  Demux/1 -> [A21]
  Demux/6 -> [A23]
  Demux/5 -> [A13]
  Demux/4 -> [A32]
  [q2] -> Gain/1
  Gain/1 -> Reciprocal/1
  Reciprocal/1 -> [q2_div]
  Add/1 -> Product/1
  [A21] -> Add/2
  [A12] -> Add/1
  [q2_div] -> Product/2
  Product/1 -> [q1]
  Product1/1 -> [q4]
  [q2_div] -> Product1/2
  [A13] -> Add1/1
  [A31] -> Add1/2
  Add1/1 -> Product1/1
  Add2/1 -> Product2/1
  [A32] -> Add2/2
  [A23] -> Add2/1
  [q2_div] -> Product2/2
  Product2/1 -> [q3]
  [q2] -> Mux/2
  [q3] -> Mux/3
  [q4] -> Mux/4

== system Quaternions_Method_main/Sun Pointing 1/Pointing error with quaternions/A_B_N from attitude det to quaternion2/If Action Subsystem2 ==
  In2 : Inport
  In1 : Inport  Port=2
  Action Port : ActionPort  ActionPortLabel=elseif( u1 == u4)
  Add : Sum  Inputs=+-
  Add1 : Sum
  Add2 : Sum  Inputs=+-
  Demux : Demux  Outputs=6
  Gain : Gain  Gain=4
  Mux : Mux
  Product : Product
  Product1 : Product
  Product2 : Product
  Reciprocal : Product  Inputs=/
  Reshape : Reshape  OutputDimensionality=Column vector (2-D)
  q_vect3 : Outport
  wires:
  [q4] -> Mux/4
  [q3] -> Mux/3
  [q2] -> Mux/2
  Product2/1 -> [q2]
  [q3_div] -> Product2/2
  [A23] -> Add2/1
  [A32] -> Add2/2
  Add2/1 -> Product2/1
  Add1/1 -> Product1/1
  [A31] -> Add1/2
  [A13] -> Add1/1
  [q3_div] -> Product1/2
  Product1/1 -> [q1]
  Product/1 -> [q4]
  [q3_div] -> Product/2
  [A12] -> Add/1
  [A21] -> Add/2
  Add/1 -> Product/1
  Reciprocal/1 -> [q3_div]
  Gain/1 -> Reciprocal/1
  [q3] -> Gain/1
  Demux/4 -> [A32]
  Demux/5 -> [A13]
  Demux/6 -> [A23]
  Demux/1 -> [A21]
  Demux/2 -> [A31]
  Demux/3 -> [A12]
  [q1] -> Mux/1
  Reshape/1 -> q_vect3/1
  Mux/1 -> Reshape/1
  In2/1 -> [q3]
  In1/1 -> Demux/1

== system Quaternions_Method_main/Sun Pointing 1/Pointing error with quaternions/A_B_N from attitude det to quaternion2/If Action Subsystem3 ==
  In2 : Inport
  In1 : Inport  Port=2
  Action Port : ActionPort  ActionPortLabel=elseif( u1 == u5)
  Add : Sum  Inputs=+-
  Add1 : Sum  Inputs=-+
  Add2 : Sum  Inputs=+-
  Demux : Demux  Outputs=6
  Gain : Gain  Gain=4
  Mux : Mux
  Product : Product
  Product1 : Product
  Product2 : Product
  Reciprocal : Product  Inputs=/
  Reshape : Reshape  OutputDimensionality=Column vector (2-D)
  q_vect4 : Outport
  wires:
  In1/1 -> Demux/1
  In2/1 -> [q4]
  Mux/1 -> Reshape/1
  Reshape/1 -> q_vect4/1
  [q1] -> Mux/1
  Demux/3 -> [A12]
  Demux/2 -> [A31]
  Demux/1 -> [A21]
  Demux/6 -> [A23]
  Demux/5 -> [A13]
  Demux/4 -> [A32]
  [q4] -> Gain/1
  Gain/1 -> Reciprocal/1
  Reciprocal/1 -> [q4_div]
  Add/1 -> Product/1
  [A21] -> Add/2
  [A12] -> Add/1
  [q4_div] -> Product/2
  Product/1 -> [q3]
  Product1/1 -> [q2]
  [q4_div] -> Product1/2
  [A13] -> Add1/1
  [A31] -> Add1/2
  Add1/1 -> Product1/1
  Add2/1 -> Product2/1
  [A32] -> Add2/2
  [A23] -> Add2/1
  [q4_div] -> Product2/2
  Product2/1 -> [q1]
  [q2] -> Mux/2
  [q3] -> Mux/3
  [q4] -> Mux/4

== system Quaternions_Method_main/Sun Pointing 1/Pointing error with quaternions/Desired attitude to quaternion1/Case 1 ==
  A11 : Inport
  A22 : Inport  Port=2
  A33 : Inport  Port=3
  Add : Sum  Inputs=++--
  Constant : Constant
  Gain : Gain  Gain=1/2
  Sqrt : Sqrt  SaturateOnIntegerOverflow=on
  q1 : Outport
  wires:
  A22/1 -> Add/3
  A11/1 -> Add/2
  A33/1 -> Add/4
  Constant/1 -> Add/1
  Add/1 -> Sqrt/1
  Sqrt/1 -> Gain/1
  Gain/1 -> q1/1

== system Quaternions_Method_main/Sun Pointing 1/Pointing error with quaternions/Desired attitude to quaternion1/Case 2 ==
  A11 : Inport
  A22 : Inport  Port=2
  A33 : Inport  Port=3
  Add : Sum  Inputs=+-+-
  Constant : Constant
  Gain : Gain  Gain=1/2
  Sqrt : Sqrt  SaturateOnIntegerOverflow=on
  q2 : Outport
  wires:
  Gain/1 -> q2/1
  Sqrt/1 -> Gain/1
  Add/1 -> Sqrt/1
  Constant/1 -> Add/1
  A33/1 -> Add/4
  A11/1 -> Add/2
  A22/1 -> Add/3

== system Quaternions_Method_main/Sun Pointing 1/Pointing error with quaternions/Desired attitude to quaternion1/Case 3 ==
  A11 : Inport
  A22 : Inport  Port=2
  A33 : Inport  Port=3
  Add : Sum  Inputs=+--+
  Constant : Constant
  Gain : Gain  Gain=1/2
  Sqrt : Sqrt  SaturateOnIntegerOverflow=on
  q3 : Outport
  wires:
  A22/1 -> Add/3
  A11/1 -> Add/2
  A33/1 -> Add/4
  Constant/1 -> Add/1
  Add/1 -> Sqrt/1
  Sqrt/1 -> Gain/1
  Gain/1 -> q3/1

== system Quaternions_Method_main/Sun Pointing 1/Pointing error with quaternions/Desired attitude to quaternion1/Case 4 ==
  A11 : Inport
  A22 : Inport  Port=2
  A33 : Inport  Port=3
  Add : Sum  Inputs=++++
  Constant : Constant
  Gain : Gain  Gain=1/2
  Sqrt : Sqrt  SaturateOnIntegerOverflow=on
  q4 : Outport
  wires:
  Gain/1 -> q4/1
  Sqrt/1 -> Gain/1
  Add/1 -> Sqrt/1
  Constant/1 -> Add/1
  A33/1 -> Add/4
  A11/1 -> Add/2
  A22/1 -> Add/3

== system Quaternions_Method_main/Sun Pointing 1/Pointing error with quaternions/Desired attitude to quaternion1/If Action Subsystem ==
  In2 : Inport
  In1 : Inport  Port=2
  Action Port : ActionPort  ActionPortLabel=if(u1 == u2)
  Add : Sum
  Add1 : Sum
  Add2 : Sum  Inputs=+-
  Demux : Demux  Outputs=6
  Gain : Gain  Gain=4
  Mux : Mux
  Product : Product
  Product1 : Product
  Product2 : Product
  Reciprocal : Product  Inputs=/
  Reshape : Reshape  OutputDimensionality=Column vector (2-D)
  q_vect1 : Outport
  wires:
  In1/1 -> Demux/1
  In2/1 -> [q1]
  Mux/1 -> Reshape/1
  Reshape/1 -> q_vect1/1
  [q1] -> Mux/1
  Demux/3 -> [A12]
  Demux/2 -> [A31]
  Demux/1 -> [A21]
  Demux/6 -> [A23]
  Demux/5 -> [A13]
  Demux/4 -> [A32]
  [q1] -> Gain/1
  Gain/1 -> Reciprocal/1
  Reciprocal/1 -> [q1_div]
  Add/1 -> Product/1
  [A21] -> Add/2
  [A12] -> Add/1
  [q1_div] -> Product/2
  Product/1 -> [q2]
  Product1/1 -> [q3]
  [q1_div] -> Product1/2
  [A13] -> Add1/1
  [A31] -> Add1/2
  Add1/1 -> Product1/1
  Add2/1 -> Product2/1
  [A32] -> Add2/2
  [A23] -> Add2/1
  [q1_div] -> Product2/2
  Product2/1 -> [q4]
  [q2] -> Mux/2
  [q3] -> Mux/3
  [q4] -> Mux/4

== system Quaternions_Method_main/Sun Pointing 1/Pointing error with quaternions/Desired attitude to quaternion1/If Action Subsystem1 ==
  In2 : Inport
  In1 : Inport  Port=2
  Action Port : ActionPort  ActionPortLabel=elseif(u1 == u3)
  Add : Sum
  Add1 : Sum  Inputs=-+
  Add2 : Sum
  Demux : Demux  Outputs=6
  Gain : Gain  Gain=4
  Mux : Mux
  Product : Product
  Product1 : Product
  Product2 : Product
  Reciprocal : Product  Inputs=/
  Reshape : Reshape  OutputDimensionality=Column vector (2-D)
  q_vect2 : Outport
  wires:
  [q4] -> Mux/4
  [q3] -> Mux/3
  [q2] -> Mux/2
  Product2/1 -> [q3]
  [q2_div] -> Product2/2
  [A23] -> Add2/1
  [A32] -> Add2/2
  Add2/1 -> Product2/1
  Add1/1 -> Product1/1
  [A31] -> Add1/2
  [A13] -> Add1/1
  [q2_div] -> Product1/2
  Product1/1 -> [q4]
  Product/1 -> [q1]
  [q2_div] -> Product/2
  [A12] -> Add/1
  [A21] -> Add/2
  Add/1 -> Product/1
  Reciprocal/1 -> [q2_div]
  Gain/1 -> Reciprocal/1
  [q2] -> Gain/1
  Demux/4 -> [A32]
  Demux/5 -> [A13]
  Demux/6 -> [A23]
  Demux/1 -> [A21]
  Demux/2 -> [A31]
  Demux/3 -> [A12]
  [q1] -> Mux/1
  Reshape/1 -> q_vect2/1
  Mux/1 -> Reshape/1
  In2/1 -> [q2]
  In1/1 -> Demux/1

== system Quaternions_Method_main/Sun Pointing 1/Pointing error with quaternions/Desired attitude to quaternion1/If Action Subsystem2 ==
  In2 : Inport
  In1 : Inport  Port=2
  Action Port : ActionPort  ActionPortLabel=elseif( u1 == u4)
  Add : Sum  Inputs=+-
  Add1 : Sum
  Add2 : Sum  Inputs=+-
  Demux : Demux  Outputs=6
  Gain : Gain  Gain=4
  Mux : Mux
  Product : Product
  Product1 : Product
  Product2 : Product
  Reciprocal : Product  Inputs=/
  Reshape : Reshape  OutputDimensionality=Column vector (2-D)
  q_vect3 : Outport
  wires:
  In1/1 -> Demux/1
  In2/1 -> [q3]
  Mux/1 -> Reshape/1
  Reshape/1 -> q_vect3/1
  [q1] -> Mux/1
  Demux/3 -> [A12]
  Demux/2 -> [A31]
  Demux/1 -> [A21]
  Demux/6 -> [A23]
  Demux/5 -> [A13]
  Demux/4 -> [A32]
  [q3] -> Gain/1
  Gain/1 -> Reciprocal/1
  Reciprocal/1 -> [q3_div]
  Add/1 -> Product/1
  [A21] -> Add/2
  [A12] -> Add/1
  [q3_div] -> Product/2
  Product/1 -> [q4]
  Product1/1 -> [q1]
  [q3_div] -> Product1/2
  [A13] -> Add1/1
  [A31] -> Add1/2
  Add1/1 -> Product1/1
  Add2/1 -> Product2/1
  [A32] -> Add2/2
  [A23] -> Add2/1
  [q3_div] -> Product2/2
  Product2/1 -> [q2]
  [q2] -> Mux/2
  [q3] -> Mux/3
  [q4] -> Mux/4

== system Quaternions_Method_main/Sun Pointing 1/Pointing error with quaternions/Desired attitude to quaternion1/If Action Subsystem3 ==
  In2 : Inport
  In1 : Inport  Port=2
  Action Port : ActionPort  ActionPortLabel=elseif( u1 == u5)
  Add : Sum  Inputs=+-
  Add1 : Sum  Inputs=-+
  Add2 : Sum  Inputs=+-
  Demux : Demux  Outputs=6
  Gain : Gain  Gain=4
  Mux : Mux
  Product : Product
  Product1 : Product
  Product2 : Product
  Reciprocal : Product  Inputs=/
  Reshape : Reshape  OutputDimensionality=Column vector (2-D)
  q_vect4 : Outport
  wires:
  [q4] -> Mux/4
  [q3] -> Mux/3
  [q2] -> Mux/2
  Product2/1 -> [q1]
  [q4_div] -> Product2/2
  [A23] -> Add2/1
  [A32] -> Add2/2
  Add2/1 -> Product2/1
  Add1/1 -> Product1/1
  [A31] -> Add1/2
  [A13] -> Add1/1
  [q4_div] -> Product1/2
  Product1/1 -> [q2]
  Product/1 -> [q3]
  [q4_div] -> Product/2
  [A12] -> Add/1
  [A21] -> Add/2
  Add/1 -> Product/1
  Reciprocal/1 -> [q4_div]
  Gain/1 -> Reciprocal/1
  [q4] -> Gain/1
  Demux/4 -> [A32]
  Demux/5 -> [A13]
  Demux/6 -> [A23]
  Demux/1 -> [A21]
  Demux/2 -> [A31]
  Demux/3 -> [A12]
  [q1] -> Mux/1
  Reshape/1 -> q_vect4/1
  Mux/1 -> Reshape/1
  In2/1 -> [q4]
  In1/1 -> Demux/1

== system Quaternions_Method_main/Enviroment/Solar Radiation Perturbation/Force1/MB Forces/Dot Product N*MB ==
  S_B : Inport
  N_MB : Inport  Port=2
  Constant3 : Constant  Value=[1, 1, 1]
  Matrix Multiply5 : Product  Multiplication=Matrix(*)
  Product10 : Product
  Reshape11 : Reshape  OutputDimensionality=Row vector (2-D)
  Reshape12 : Reshape  OutputDimensionality=Column vector (2-D)
  Sum of Elements : Sum  Inputs=+  CollapseMode=Specified dimension  CollapseDim=2
  Out1 : Outport
  wires:
  N_MB/1 -> Product10/2
  Reshape11/1 -> Matrix Multiply5/1
  Constant3/1 -> Reshape11/1
  Matrix Multiply5/1 -> Product10/1
  Sum of Elements/1 -> Out1/1
  S_B/1 -> Reshape12/1
  Reshape12/1 -> Matrix Multiply5/2
  Product10/1 -> Sum of Elements/1

== system Quaternions_Method_main/Enviroment/Solar Radiation Perturbation/Force1/MB Forces/creation of the areas of the S//C ==
  note: creation of areas of MB:
      | a=lato corto su asse x del BF; b=lato lungo lungo asse y del BF; h = spessore lungo asse z del BF
  MB : Inport
  Demux : Demux
  Product1 : Product
  Product2 : Product
  Product4 : Product
  Terminator : Terminator
  a*b_1 : Outport
  a*b_2 : Outport  Port=2
  a*h_1 : Outport  Port=3
  a*h_2 : Outport  Port=4
  b*h_1 : Outport  Port=5
  b*h_2 : Outport  Port=6
  wires:
  Demux/4 -> Product4/1, Product2/2
  Demux/3 -> Product1/2, Product4/2
  Demux/2 -> Product1/1, Product2/1
  Product1/1 -> a*b_2/1, a*b_1/1  "a*b"
  Product2/1 -> a*h_1/1, a*h_2/1  "a*h"
  Product4/1 -> b*h_2/1, b*h_1/1  "b*h"
  MB/1 -> Demux/1
  Demux/1 -> Terminator/1

== system Quaternions_Method_main/Enviroment/Solar Radiation Perturbation/Force1/SP Forces/Dot Product N*SP ==
  S_B : Inport
  N_SP : Inport  Port=2
  Constant11 : Constant  Value=[1, 1, 1]
  Matrix Multiply7 : Product  Multiplication=Matrix(*)
  Product11 : Product
  Reshape13 : Reshape  OutputDimensionality=Column vector (2-D)
  Reshape8 : Reshape  OutputDimensionality=Row vector (2-D)
  Sum of Elements1 : Sum  Inputs=+  CollapseMode=Specified dimension  CollapseDim=2
  dot_N_SP_SB : Outport
  wires:
  Reshape13/1 -> Matrix Multiply7/2
  Matrix Multiply7/1 -> Product11/1
  N_SP/1 -> Product11/2
  Constant11/1 -> Reshape8/1
  Product11/1 -> Sum of Elements1/1
  Reshape8/1 -> Matrix Multiply7/1
  Sum of Elements1/1 -> dot_N_SP_SB/1
  S_B/1 -> Reshape13/1

== system Quaternions_Method_main/Enviroment/Solar Radiation Perturbation/Force1/SP Forces/creation of the areas of the S//C ==
  note: creation of areas of SP:
      | a=lato corto su asse x del BF; b=lato lungo lungo asse y del BF;
      | lato h è trascurabile
      | il procedimento è per 2 pannelli quindi in tutto ho 4 facce
  SP : Inport
  Demux1 : Demux
  Product1 : Product
  Terminator1 : Terminator
  Terminator3 : Terminator
  a*b_1 : Outport
  a*b_2 : Outport  Port=2
  a*b_3 : Outport  Port=3
  a*b_4 : Outport  Port=4
  wires:
  SP/1 -> Demux1/1
  Demux1/1 -> Terminator1/1
  Demux1/4 -> Terminator3/1
  Demux1/3 -> Product1/2
  Product1/1 -> a*b_3/1, a*b_1/1, a*b_4/1, a*b_2/1  "a*b"
  Demux1/2 -> Product1/1

== system Quaternions_Method_main/Enviroment/Solar Radiation Perturbation/Sum forces/determine highlighted area/If Action Subsystem ==
  In1 : Inport
  Action Port : ActionPort  ActionPortLabel=if(u1>0 )
  Out1 : Outport
  wires:
  In1/1 -> Out1/1

== system Quaternions_Method_main/Enviroment/Solar Radiation Perturbation/Sum forces/determine highlighted area/If Action Subsystem1 ==
  In1 : Inport
  Action Port : ActionPort  ActionPortLabel=elseif(u2>0)
  Out1 : Outport
  wires:
  In1/1 -> Out1/1

== system Quaternions_Method_main/Enviroment/Solar Radiation Perturbation/Sum forces/determine highlighted area/If Action Subsystem2 ==
  Action Port : ActionPort  ActionPortLabel=else
  Constant : Constant  Value=0
  Out1 : Outport
  wires:
  Constant/1 -> Out1/1

== system Quaternions_Method_main/Enviroment/Solar Radiation Perturbation/Sum forces/determine highlighted area/If Action Subsystem3 ==
  In1 : Inport
  Action Port : ActionPort  ActionPortLabel=if(u1>0 )
  Out1 : Outport
  wires:
  In1/1 -> Out1/1

== system Quaternions_Method_main/Enviroment/Solar Radiation Perturbation/Sum forces/determine highlighted area/If Action Subsystem4 ==
  In1 : Inport
  Action Port : ActionPort  ActionPortLabel=elseif(u2>0)
  Out1 : Outport
  wires:
  In1/1 -> Out1/1

== system Quaternions_Method_main/Enviroment/Solar Radiation Perturbation/Sum forces/determine highlighted area/If Action Subsystem5 ==
  Action Port : ActionPort  ActionPortLabel=else
  Constant : Constant  Value=0
  Out1 : Outport
  wires:
  Constant/1 -> Out1/1

== system Quaternions_Method_main/Enviroment/Solar Radiation Perturbation/Sum forces/determine highlighted area/If Action Subsystem6 ==
  In1 : Inport
  Action Port : ActionPort  ActionPortLabel=if(u1>0 )
  Out1 : Outport
  wires:
  In1/1 -> Out1/1

== system Quaternions_Method_main/Enviroment/Solar Radiation Perturbation/Sum forces/determine highlighted area/If Action Subsystem7 ==
  In1 : Inport
  Action Port : ActionPort  ActionPortLabel=elseif(u2>0)
  Out1 : Outport
  wires:
  In1/1 -> Out1/1

== system Quaternions_Method_main/Enviroment/Solar Radiation Perturbation/Sum forces/determine highlighted area/If Action Subsystem8 ==
  Action Port : ActionPort  ActionPortLabel=else
  Constant : Constant  Value=0
  Out1 : Outport
  wires:
  Constant/1 -> Out1/1
